simulink model "gm_parallel_lht"  (R2019b)
settings: Solver=FixedStepDiscrete  StartTime=0.0  StopTime=inf  RelTol=1e-3
undefined symbols (not defined in the file or in its folder): bt, height, width
libraries: hdlsllib x190, simulink x13, hdlmdlgenlib x7, dspsrcs4 x1
(part 11 of 18)

== system gm_parallel_lht/Parallel LHT/Parallel LHT Accumulator/Accumulator with Switches/Accumulator_instance41/Block RAM ==
  wr_data : Inport  OutDataTypeStr=fixdt(0, 10, 0)  PortDimensions=1  SampleTime=6.66666666666667e-09
  wr_addr : Inport  Port=2  OutDataTypeStr=fixdt(0, 10, 0)  PortDimensions=1  SampleTime=6.66666666666667e-09
  wr_en : Inport  Port=3  OutDataTypeStr=boolean  PortDimensions=1  SampleTime=6.66666666666667e-09
  rd_addr : Inport  Port=4  OutDataTypeStr=fixdt(0, 10, 0)  PortDimensions=1  SampleTime=6.66666666666667e-09
  Simple Dual Port RAM : Subsystem
  rd_data : Outport
  wires:
  rd_addr/1 -> Simple Dual Port RAM/4(rd_addr)
  wr_en/1 -> Simple Dual Port RAM/3(wr_en)
  wr_addr/1 -> Simple Dual Port RAM/2(wr_addr)
  wr_data/1 -> Simple Dual Port RAM/1(wr_data)
  Simple Dual Port RAM/1(rd_data) -> rd_data/1

== system gm_parallel_lht/Parallel LHT/Parallel LHT Accumulator/Accumulator with Switches/Accumulator_instance42/Block RAM ==
  wr_data : Inport  OutDataTypeStr=fixdt(0, 10, 0)  PortDimensions=1  SampleTime=6.66666666666667e-09
  wr_addr : Inport  Port=2  OutDataTypeStr=fixdt(0, 10, 0)  PortDimensions=1  SampleTime=6.66666666666667e-09
  wr_en : Inport  Port=3  OutDataTypeStr=boolean  PortDimensions=1  SampleTime=6.66666666666667e-09
  rd_addr : Inport  Port=4  OutDataTypeStr=fixdt(0, 10, 0)  PortDimensions=1  SampleTime=6.66666666666667e-09
  Simple Dual Port RAM : Subsystem
  rd_data : Outport
  wires:
  rd_addr/1 -> Simple Dual Port RAM/4(rd_addr)
  wr_en/1 -> Simple Dual Port RAM/3(wr_en)
  wr_addr/1 -> Simple Dual Port RAM/2(wr_addr)
  wr_data/1 -> Simple Dual Port RAM/1(wr_data)
  Simple Dual Port RAM/1(rd_data) -> rd_data/1

== system gm_parallel_lht/Parallel LHT/Parallel LHT Accumulator/Accumulator with Switches/Accumulator_instance43/Block RAM ==
  wr_data : Inport  OutDataTypeStr=fixdt(0, 10, 0)  PortDimensions=1  SampleTime=6.66666666666667e-09
  wr_addr : Inport  Port=2  OutDataTypeStr=fixdt(0, 10, 0)  PortDimensions=1  SampleTime=6.66666666666667e-09
  wr_en : Inport  Port=3  OutDataTypeStr=boolean  PortDimensions=1  SampleTime=6.66666666666667e-09
  rd_addr : Inport  Port=4  OutDataTypeStr=fixdt(0, 10, 0)  PortDimensions=1  SampleTime=6.66666666666667e-09
  Simple Dual Port RAM : Subsystem
  rd_data : Outport
  wires:
  rd_addr/1 -> Simple Dual Port RAM/4(rd_addr)
  wr_en/1 -> Simple Dual Port RAM/3(wr_en)
  wr_addr/1 -> Simple Dual Port RAM/2(wr_addr)
  wr_data/1 -> Simple Dual Port RAM/1(wr_data)
  Simple Dual Port RAM/1(rd_data) -> rd_data/1

== system gm_parallel_lht/Parallel LHT/Parallel LHT Accumulator/Accumulator with Switches/Accumulator_instance44/Block RAM ==
  wr_data : Inport  OutDataTypeStr=fixdt(0, 10, 0)  PortDimensions=1  SampleTime=6.66666666666667e-09
  wr_addr : Inport  Port=2  OutDataTypeStr=fixdt(0, 10, 0)  PortDimensions=1  SampleTime=6.66666666666667e-09
  wr_en : Inport  Port=3  OutDataTypeStr=boolean  PortDimensions=1  SampleTime=6.66666666666667e-09
  rd_addr : Inport  Port=4  OutDataTypeStr=fixdt(0, 10, 0)  PortDimensions=1  SampleTime=6.66666666666667e-09
  Simple Dual Port RAM : Subsystem
  rd_data : Outport
  wires:
  rd_addr/1 -> Simple Dual Port RAM/4(rd_addr)
  wr_en/1 -> Simple Dual Port RAM/3(wr_en)
  wr_addr/1 -> Simple Dual Port RAM/2(wr_addr)
  wr_data/1 -> Simple Dual Port RAM/1(wr_data)
  Simple Dual Port RAM/1(rd_data) -> rd_data/1

== system gm_parallel_lht/Parallel LHT/Parallel LHT Accumulator/Accumulator with Switches/Accumulator_instance45/Block RAM ==
  wr_data : Inport  OutDataTypeStr=fixdt(0, 10, 0)  PortDimensions=1  SampleTime=6.66666666666667e-09
  wr_addr : Inport  Port=2  OutDataTypeStr=fixdt(0, 10, 0)  PortDimensions=1  SampleTime=6.66666666666667e-09
  wr_en : Inport  Port=3  OutDataTypeStr=boolean  PortDimensions=1  SampleTime=6.66666666666667e-09
  rd_addr : Inport  Port=4  OutDataTypeStr=fixdt(0, 10, 0)  PortDimensions=1  SampleTime=6.66666666666667e-09
  Simple Dual Port RAM : Subsystem
  rd_data : Outport
  wires:
  rd_addr/1 -> Simple Dual Port RAM/4(rd_addr)
  wr_en/1 -> Simple Dual Port RAM/3(wr_en)
  wr_addr/1 -> Simple Dual Port RAM/2(wr_addr)
  wr_data/1 -> Simple Dual Port RAM/1(wr_data)
  Simple Dual Port RAM/1(rd_data) -> rd_data/1

== system gm_parallel_lht/Parallel LHT/Parallel LHT Accumulator/Accumulator with Switches/Accumulator_instance46/Block RAM ==
  wr_data : Inport  OutDataTypeStr=fixdt(0, 10, 0)  PortDimensions=1  SampleTime=6.66666666666667e-09
  wr_addr : Inport  Port=2  OutDataTypeStr=fixdt(0, 10, 0)  PortDimensions=1  SampleTime=6.66666666666667e-09
  wr_en : Inport  Port=3  OutDataTypeStr=boolean  PortDimensions=1  SampleTime=6.66666666666667e-09
  rd_addr : Inport  Port=4  OutDataTypeStr=fixdt(0, 10, 0)  PortDimensions=1  SampleTime=6.66666666666667e-09
  Simple Dual Port RAM : Subsystem
  rd_data : Outport
  wires:
  rd_addr/1 -> Simple Dual Port RAM/4(rd_addr)
  wr_en/1 -> Simple Dual Port RAM/3(wr_en)
  wr_addr/1 -> Simple Dual Port RAM/2(wr_addr)
  wr_data/1 -> Simple Dual Port RAM/1(wr_data)
  Simple Dual Port RAM/1(rd_data) -> rd_data/1

== system gm_parallel_lht/Parallel LHT/Parallel LHT Accumulator/Accumulator with Switches/Accumulator_instance47/Block RAM ==
  wr_data : Inport  OutDataTypeStr=fixdt(0, 10, 0)  PortDimensions=1  SampleTime=6.66666666666667e-09
  wr_addr : Inport  Port=2  OutDataTypeStr=fixdt(0, 10, 0)  PortDimensions=1  SampleTime=6.66666666666667e-09
  wr_en : Inport  Port=3  OutDataTypeStr=boolean  PortDimensions=1  SampleTime=6.66666666666667e-09
  rd_addr : Inport  Port=4  OutDataTypeStr=fixdt(0, 10, 0)  PortDimensions=1  SampleTime=6.66666666666667e-09
  Simple Dual Port RAM : Subsystem
  rd_data : Outport
  wires:
  rd_addr/1 -> Simple Dual Port RAM/4(rd_addr)
  wr_en/1 -> Simple Dual Port RAM/3(wr_en)
  wr_addr/1 -> Simple Dual Port RAM/2(wr_addr)
  wr_data/1 -> Simple Dual Port RAM/1(wr_data)
  Simple Dual Port RAM/1(rd_data) -> rd_data/1

== system gm_parallel_lht/Parallel LHT/Parallel LHT Accumulator/Accumulator with Switches/Accumulator_instance48/Block RAM ==
  wr_data : Inport  OutDataTypeStr=fixdt(0, 10, 0)  PortDimensions=1  SampleTime=6.66666666666667e-09
  wr_addr : Inport  Port=2  OutDataTypeStr=fixdt(0, 10, 0)  PortDimensions=1  SampleTime=6.66666666666667e-09
  wr_en : Inport  Port=3  OutDataTypeStr=boolean  PortDimensions=1  SampleTime=6.66666666666667e-09
  rd_addr : Inport  Port=4  OutDataTypeStr=fixdt(0, 10, 0)  PortDimensions=1  SampleTime=6.66666666666667e-09
  Simple Dual Port RAM : Subsystem
  rd_data : Outport
  wires:
  rd_addr/1 -> Simple Dual Port RAM/4(rd_addr)
  wr_en/1 -> Simple Dual Port RAM/3(wr_en)
  wr_addr/1 -> Simple Dual Port RAM/2(wr_addr)
  wr_data/1 -> Simple Dual Port RAM/1(wr_data)
  Simple Dual Port RAM/1(rd_data) -> rd_data/1

== system gm_parallel_lht/Parallel LHT/Parallel LHT Accumulator/Accumulator with Switches/Accumulator_instance49/Block RAM ==
  wr_data : Inport  OutDataTypeStr=fixdt(0, 10, 0)  PortDimensions=1  SampleTime=6.66666666666667e-09
  wr_addr : Inport  Port=2  OutDataTypeStr=fixdt(0, 10, 0)  PortDimensions=1  SampleTime=6.66666666666667e-09
  wr_en : Inport  Port=3  OutDataTypeStr=boolean  PortDimensions=1  SampleTime=6.66666666666667e-09
  rd_addr : Inport  Port=4  OutDataTypeStr=fixdt(0, 10, 0)  PortDimensions=1  SampleTime=6.66666666666667e-09
  Simple Dual Port RAM : Subsystem
  rd_data : Outport
  wires:
  rd_addr/1 -> Simple Dual Port RAM/4(rd_addr)
  wr_en/1 -> Simple Dual Port RAM/3(wr_en)
  wr_addr/1 -> Simple Dual Port RAM/2(wr_addr)
  wr_data/1 -> Simple Dual Port RAM/1(wr_data)
  Simple Dual Port RAM/1(rd_data) -> rd_data/1

== system gm_parallel_lht/Parallel LHT/Parallel LHT Accumulator/Accumulator with Switches/Accumulator_instance5/Block RAM ==
  wr_data : Inport  OutDataTypeStr=fixdt(0, 10, 0)  PortDimensions=1  SampleTime=6.66666666666667e-09
  wr_addr : Inport  Port=2  OutDataTypeStr=fixdt(0, 10, 0)  PortDimensions=1  SampleTime=6.66666666666667e-09
  wr_en : Inport  Port=3  OutDataTypeStr=boolean  PortDimensions=1  SampleTime=6.66666666666667e-09
  rd_addr : Inport  Port=4  OutDataTypeStr=fixdt(0, 10, 0)  PortDimensions=1  SampleTime=6.66666666666667e-09
  Simple Dual Port RAM : Subsystem
  rd_data : Outport
  wires:
  rd_addr/1 -> Simple Dual Port RAM/4(rd_addr)
  wr_en/1 -> Simple Dual Port RAM/3(wr_en)
  wr_addr/1 -> Simple Dual Port RAM/2(wr_addr)
  wr_data/1 -> Simple Dual Port RAM/1(wr_data)
  Simple Dual Port RAM/1(rd_data) -> rd_data/1

== system gm_parallel_lht/Parallel LHT/Parallel LHT Accumulator/Accumulator with Switches/Accumulator_instance50/Block RAM ==
  wr_data : Inport  OutDataTypeStr=fixdt(0, 10, 0)  PortDimensions=1  SampleTime=6.66666666666667e-09
  wr_addr : Inport  Port=2  OutDataTypeStr=fixdt(0, 10, 0)  PortDimensions=1  SampleTime=6.66666666666667e-09
  wr_en : Inport  Port=3  OutDataTypeStr=boolean  PortDimensions=1  SampleTime=6.66666666666667e-09
  rd_addr : Inport  Port=4  OutDataTypeStr=fixdt(0, 10, 0)  PortDimensions=1  SampleTime=6.66666666666667e-09
  Simple Dual Port RAM : Subsystem
  rd_data : Outport
  wires:
  rd_addr/1 -> Simple Dual Port RAM/4(rd_addr)
  wr_en/1 -> Simple Dual Port RAM/3(wr_en)
  wr_addr/1 -> Simple Dual Port RAM/2(wr_addr)
  wr_data/1 -> Simple Dual Port RAM/1(wr_data)
  Simple Dual Port RAM/1(rd_data) -> rd_data/1

== system gm_parallel_lht/Parallel LHT/Parallel LHT Accumulator/Accumulator with Switches/Accumulator_instance51/Block RAM ==
  wr_data : Inport  OutDataTypeStr=fixdt(0, 10, 0)  PortDimensions=1  SampleTime=6.66666666666667e-09
  wr_addr : Inport  Port=2  OutDataTypeStr=fixdt(0, 10, 0)  PortDimensions=1  SampleTime=6.66666666666667e-09
  wr_en : Inport  Port=3  OutDataTypeStr=boolean  PortDimensions=1  SampleTime=6.66666666666667e-09
  rd_addr : Inport  Port=4  OutDataTypeStr=fixdt(0, 10, 0)  PortDimensions=1  SampleTime=6.66666666666667e-09
  Simple Dual Port RAM : Subsystem
  rd_data : Outport
  wires:
  rd_addr/1 -> Simple Dual Port RAM/4(rd_addr)
  wr_en/1 -> Simple Dual Port RAM/3(wr_en)
  wr_addr/1 -> Simple Dual Port RAM/2(wr_addr)
  wr_data/1 -> Simple Dual Port RAM/1(wr_data)
  Simple Dual Port RAM/1(rd_data) -> rd_data/1

== system gm_parallel_lht/Parallel LHT/Parallel LHT Accumulator/Accumulator with Switches/Accumulator_instance52/Block RAM ==
  wr_data : Inport  OutDataTypeStr=fixdt(0, 10, 0)  PortDimensions=1  SampleTime=6.66666666666667e-09
  wr_addr : Inport  Port=2  OutDataTypeStr=fixdt(0, 10, 0)  PortDimensions=1  SampleTime=6.66666666666667e-09
  wr_en : Inport  Port=3  OutDataTypeStr=boolean  PortDimensions=1  SampleTime=6.66666666666667e-09
  rd_addr : Inport  Port=4  OutDataTypeStr=fixdt(0, 10, 0)  PortDimensions=1  SampleTime=6.66666666666667e-09
  Simple Dual Port RAM : Subsystem
  rd_data : Outport
  wires:
  rd_addr/1 -> Simple Dual Port RAM/4(rd_addr)
  wr_en/1 -> Simple Dual Port RAM/3(wr_en)
  wr_addr/1 -> Simple Dual Port RAM/2(wr_addr)
  wr_data/1 -> Simple Dual Port RAM/1(wr_data)
  Simple Dual Port RAM/1(rd_data) -> rd_data/1

== system gm_parallel_lht/Parallel LHT/Parallel LHT Accumulator/Accumulator with Switches/Accumulator_instance53/Block RAM ==
  wr_data : Inport  OutDataTypeStr=fixdt(0, 10, 0)  PortDimensions=1  SampleTime=6.66666666666667e-09
  wr_addr : Inport  Port=2  OutDataTypeStr=fixdt(0, 10, 0)  PortDimensions=1  SampleTime=6.66666666666667e-09
  wr_en : Inport  Port=3  OutDataTypeStr=boolean  PortDimensions=1  SampleTime=6.66666666666667e-09
  rd_addr : Inport  Port=4  OutDataTypeStr=fixdt(0, 10, 0)  PortDimensions=1  SampleTime=6.66666666666667e-09
  Simple Dual Port RAM : Subsystem
  rd_data : Outport
  wires:
  rd_addr/1 -> Simple Dual Port RAM/4(rd_addr)
  wr_en/1 -> Simple Dual Port RAM/3(wr_en)
  wr_addr/1 -> Simple Dual Port RAM/2(wr_addr)
  wr_data/1 -> Simple Dual Port RAM/1(wr_data)
  Simple Dual Port RAM/1(rd_data) -> rd_data/1

== system gm_parallel_lht/Parallel LHT/Parallel LHT Accumulator/Accumulator with Switches/Accumulator_instance54/Block RAM ==
  wr_data : Inport  OutDataTypeStr=fixdt(0, 10, 0)  PortDimensions=1  SampleTime=6.66666666666667e-09
  wr_addr : Inport  Port=2  OutDataTypeStr=fixdt(0, 10, 0)  PortDimensions=1  SampleTime=6.66666666666667e-09
  wr_en : Inport  Port=3  OutDataTypeStr=boolean  PortDimensions=1  SampleTime=6.66666666666667e-09
  rd_addr : Inport  Port=4  OutDataTypeStr=fixdt(0, 10, 0)  PortDimensions=1  SampleTime=6.66666666666667e-09
  Simple Dual Port RAM : Subsystem
  rd_data : Outport
  wires:
  rd_addr/1 -> Simple Dual Port RAM/4(rd_addr)
  wr_en/1 -> Simple Dual Port RAM/3(wr_en)
  wr_addr/1 -> Simple Dual Port RAM/2(wr_addr)
  wr_data/1 -> Simple Dual Port RAM/1(wr_data)
  Simple Dual Port RAM/1(rd_data) -> rd_data/1

== system gm_parallel_lht/Parallel LHT/Parallel LHT Accumulator/Accumulator with Switches/Accumulator_instance55/Block RAM ==
  wr_data : Inport  OutDataTypeStr=fixdt(0, 10, 0)  PortDimensions=1  SampleTime=6.66666666666667e-09
  wr_addr : Inport  Port=2  OutDataTypeStr=fixdt(0, 10, 0)  PortDimensions=1  SampleTime=6.66666666666667e-09
  wr_en : Inport  Port=3  OutDataTypeStr=boolean  PortDimensions=1  SampleTime=6.66666666666667e-09
  rd_addr : Inport  Port=4  OutDataTypeStr=fixdt(0, 10, 0)  PortDimensions=1  SampleTime=6.66666666666667e-09
  Simple Dual Port RAM : Subsystem
  rd_data : Outport
  wires:
  rd_addr/1 -> Simple Dual Port RAM/4(rd_addr)
  wr_en/1 -> Simple Dual Port RAM/3(wr_en)
  wr_addr/1 -> Simple Dual Port RAM/2(wr_addr)
  wr_data/1 -> Simple Dual Port RAM/1(wr_data)
  Simple Dual Port RAM/1(rd_data) -> rd_data/1

== system gm_parallel_lht/Parallel LHT/Parallel LHT Accumulator/Accumulator with Switches/Accumulator_instance56/Block RAM ==
  wr_data : Inport  OutDataTypeStr=fixdt(0, 10, 0)  PortDimensions=1  SampleTime=6.66666666666667e-09
  wr_addr : Inport  Port=2  OutDataTypeStr=fixdt(0, 10, 0)  PortDimensions=1  SampleTime=6.66666666666667e-09
  wr_en : Inport  Port=3  OutDataTypeStr=boolean  PortDimensions=1  SampleTime=6.66666666666667e-09
  rd_addr : Inport  Port=4  OutDataTypeStr=fixdt(0, 10, 0)  PortDimensions=1  SampleTime=6.66666666666667e-09
  Simple Dual Port RAM : Subsystem
  rd_data : Outport
  wires:
  rd_addr/1 -> Simple Dual Port RAM/4(rd_addr)
  wr_en/1 -> Simple Dual Port RAM/3(wr_en)
  wr_addr/1 -> Simple Dual Port RAM/2(wr_addr)
  wr_data/1 -> Simple Dual Port RAM/1(wr_data)
  Simple Dual Port RAM/1(rd_data) -> rd_data/1

== system gm_parallel_lht/Parallel LHT/Parallel LHT Accumulator/Accumulator with Switches/Accumulator_instance57/Block RAM ==
  wr_data : Inport  OutDataTypeStr=fixdt(0, 10, 0)  PortDimensions=1  SampleTime=6.66666666666667e-09
  wr_addr : Inport  Port=2  OutDataTypeStr=fixdt(0, 10, 0)  PortDimensions=1  SampleTime=6.66666666666667e-09
  wr_en : Inport  Port=3  OutDataTypeStr=boolean  PortDimensions=1  SampleTime=6.66666666666667e-09
  rd_addr : Inport  Port=4  OutDataTypeStr=fixdt(0, 10, 0)  PortDimensions=1  SampleTime=6.66666666666667e-09
  Simple Dual Port RAM : Subsystem
  rd_data : Outport
  wires:
  rd_addr/1 -> Simple Dual Port RAM/4(rd_addr)
  wr_en/1 -> Simple Dual Port RAM/3(wr_en)
  wr_addr/1 -> Simple Dual Port RAM/2(wr_addr)
  wr_data/1 -> Simple Dual Port RAM/1(wr_data)
  Simple Dual Port RAM/1(rd_data) -> rd_data/1

== system gm_parallel_lht/Parallel LHT/Parallel LHT Accumulator/Accumulator with Switches/Accumulator_instance58/Block RAM ==
  wr_data : Inport  OutDataTypeStr=fixdt(0, 10, 0)  PortDimensions=1  SampleTime=6.66666666666667e-09
  wr_addr : Inport  Port=2  OutDataTypeStr=fixdt(0, 10, 0)  PortDimensions=1  SampleTime=6.66666666666667e-09
  wr_en : Inport  Port=3  OutDataTypeStr=boolean  PortDimensions=1  SampleTime=6.66666666666667e-09
  rd_addr : Inport  Port=4  OutDataTypeStr=fixdt(0, 10, 0)  PortDimensions=1  SampleTime=6.66666666666667e-09
  Simple Dual Port RAM : Subsystem
  rd_data : Outport
  wires:
  rd_addr/1 -> Simple Dual Port RAM/4(rd_addr)
  wr_en/1 -> Simple Dual Port RAM/3(wr_en)
  wr_addr/1 -> Simple Dual Port RAM/2(wr_addr)
  wr_data/1 -> Simple Dual Port RAM/1(wr_data)
  Simple Dual Port RAM/1(rd_data) -> rd_data/1

== system gm_parallel_lht/Parallel LHT/Parallel LHT Accumulator/Accumulator with Switches/Accumulator_instance59/Block RAM ==
  wr_data : Inport  OutDataTypeStr=fixdt(0, 10, 0)  PortDimensions=1  SampleTime=6.66666666666667e-09
  wr_addr : Inport  Port=2  OutDataTypeStr=fixdt(0, 10, 0)  PortDimensions=1  SampleTime=6.66666666666667e-09
  wr_en : Inport  Port=3  OutDataTypeStr=boolean  PortDimensions=1  SampleTime=6.66666666666667e-09
  rd_addr : Inport  Port=4  OutDataTypeStr=fixdt(0, 10, 0)  PortDimensions=1  SampleTime=6.66666666666667e-09
  Simple Dual Port RAM : Subsystem
  rd_data : Outport
  wires:
  rd_addr/1 -> Simple Dual Port RAM/4(rd_addr)
  wr_en/1 -> Simple Dual Port RAM/3(wr_en)
  wr_addr/1 -> Simple Dual Port RAM/2(wr_addr)
  wr_data/1 -> Simple Dual Port RAM/1(wr_data)
  Simple Dual Port RAM/1(rd_data) -> rd_data/1

== system gm_parallel_lht/Parallel LHT/Parallel LHT Accumulator/Accumulator with Switches/Accumulator_instance6/Block RAM ==
  wr_data : Inport  OutDataTypeStr=fixdt(0, 10, 0)  PortDimensions=1  SampleTime=6.66666666666667e-09
  wr_addr : Inport  Port=2  OutDataTypeStr=fixdt(0, 10, 0)  PortDimensions=1  SampleTime=6.66666666666667e-09
  wr_en : Inport  Port=3  OutDataTypeStr=boolean  PortDimensions=1  SampleTime=6.66666666666667e-09
  rd_addr : Inport  Port=4  OutDataTypeStr=fixdt(0, 10, 0)  PortDimensions=1  SampleTime=6.66666666666667e-09
  Simple Dual Port RAM : Subsystem
  rd_data : Outport
  wires:
  rd_addr/1 -> Simple Dual Port RAM/4(rd_addr)
  wr_en/1 -> Simple Dual Port RAM/3(wr_en)
  wr_addr/1 -> Simple Dual Port RAM/2(wr_addr)
  wr_data/1 -> Simple Dual Port RAM/1(wr_data)
  Simple Dual Port RAM/1(rd_data) -> rd_data/1

== system gm_parallel_lht/Parallel LHT/Parallel LHT Accumulator/Accumulator with Switches/Accumulator_instance60/Block RAM ==
  wr_data : Inport  OutDataTypeStr=fixdt(0, 10, 0)  PortDimensions=1  SampleTime=6.66666666666667e-09
  wr_addr : Inport  Port=2  OutDataTypeStr=fixdt(0, 10, 0)  PortDimensions=1  SampleTime=6.66666666666667e-09
  wr_en : Inport  Port=3  OutDataTypeStr=boolean  PortDimensions=1  SampleTime=6.66666666666667e-09
  rd_addr : Inport  Port=4  OutDataTypeStr=fixdt(0, 10, 0)  PortDimensions=1  SampleTime=6.66666666666667e-09
  Simple Dual Port RAM : Subsystem
  rd_data : Outport
  wires:
  rd_addr/1 -> Simple Dual Port RAM/4(rd_addr)
  wr_en/1 -> Simple Dual Port RAM/3(wr_en)
  wr_addr/1 -> Simple Dual Port RAM/2(wr_addr)
  wr_data/1 -> Simple Dual Port RAM/1(wr_data)
  Simple Dual Port RAM/1(rd_data) -> rd_data/1

== system gm_parallel_lht/Parallel LHT/Parallel LHT Accumulator/Accumulator with Switches/Accumulator_instance61/Block RAM ==
  wr_data : Inport  OutDataTypeStr=fixdt(0, 10, 0)  PortDimensions=1  SampleTime=6.66666666666667e-09
  wr_addr : Inport  Port=2  OutDataTypeStr=fixdt(0, 10, 0)  PortDimensions=1  SampleTime=6.66666666666667e-09
  wr_en : Inport  Port=3  OutDataTypeStr=boolean  PortDimensions=1  SampleTime=6.66666666666667e-09
  rd_addr : Inport  Port=4  OutDataTypeStr=fixdt(0, 10, 0)  PortDimensions=1  SampleTime=6.66666666666667e-09
  Simple Dual Port RAM : Subsystem
  rd_data : Outport
  wires:
  rd_addr/1 -> Simple Dual Port RAM/4(rd_addr)
  wr_en/1 -> Simple Dual Port RAM/3(wr_en)
  wr_addr/1 -> Simple Dual Port RAM/2(wr_addr)
  wr_data/1 -> Simple Dual Port RAM/1(wr_data)
  Simple Dual Port RAM/1(rd_data) -> rd_data/1

== system gm_parallel_lht/Parallel LHT/Parallel LHT Accumulator/Accumulator with Switches/Accumulator_instance62/Block RAM ==
  wr_data : Inport  OutDataTypeStr=fixdt(0, 10, 0)  PortDimensions=1  SampleTime=6.66666666666667e-09
  wr_addr : Inport  Port=2  OutDataTypeStr=fixdt(0, 10, 0)  PortDimensions=1  SampleTime=6.66666666666667e-09
  wr_en : Inport  Port=3  OutDataTypeStr=boolean  PortDimensions=1  SampleTime=6.66666666666667e-09
  rd_addr : Inport  Port=4  OutDataTypeStr=fixdt(0, 10, 0)  PortDimensions=1  SampleTime=6.66666666666667e-09
  Simple Dual Port RAM : Subsystem
  rd_data : Outport
  wires:
  rd_addr/1 -> Simple Dual Port RAM/4(rd_addr)
  wr_en/1 -> Simple Dual Port RAM/3(wr_en)
  wr_addr/1 -> Simple Dual Port RAM/2(wr_addr)
  wr_data/1 -> Simple Dual Port RAM/1(wr_data)
  Simple Dual Port RAM/1(rd_data) -> rd_data/1

== system gm_parallel_lht/Parallel LHT/Parallel LHT Accumulator/Accumulator with Switches/Accumulator_instance63/Block RAM ==
  wr_data : Inport  OutDataTypeStr=fixdt(0, 10, 0)  PortDimensions=1  SampleTime=6.66666666666667e-09
  wr_addr : Inport  Port=2  OutDataTypeStr=fixdt(0, 10, 0)  PortDimensions=1  SampleTime=6.66666666666667e-09
  wr_en : Inport  Port=3  OutDataTypeStr=boolean  PortDimensions=1  SampleTime=6.66666666666667e-09
  rd_addr : Inport  Port=4  OutDataTypeStr=fixdt(0, 10, 0)  PortDimensions=1  SampleTime=6.66666666666667e-09
  Simple Dual Port RAM : Subsystem
  rd_data : Outport
  wires:
  rd_addr/1 -> Simple Dual Port RAM/4(rd_addr)
  wr_en/1 -> Simple Dual Port RAM/3(wr_en)
  wr_addr/1 -> Simple Dual Port RAM/2(wr_addr)
  wr_data/1 -> Simple Dual Port RAM/1(wr_data)
  Simple Dual Port RAM/1(rd_data) -> rd_data/1

== system gm_parallel_lht/Parallel LHT/Parallel LHT Accumulator/Accumulator with Switches/Accumulator_instance64/Block RAM ==
  wr_data : Inport  OutDataTypeStr=fixdt(0, 10, 0)  PortDimensions=1  SampleTime=6.66666666666667e-09
  wr_addr : Inport  Port=2  OutDataTypeStr=fixdt(0, 10, 0)  PortDimensions=1  SampleTime=6.66666666666667e-09
  wr_en : Inport  Port=3  OutDataTypeStr=boolean  PortDimensions=1  SampleTime=6.66666666666667e-09
  rd_addr : Inport  Port=4  OutDataTypeStr=fixdt(0, 10, 0)  PortDimensions=1  SampleTime=6.66666666666667e-09
  Simple Dual Port RAM : Subsystem
  rd_data : Outport
  wires:
  rd_addr/1 -> Simple Dual Port RAM/4(rd_addr)
  wr_en/1 -> Simple Dual Port RAM/3(wr_en)
  wr_addr/1 -> Simple Dual Port RAM/2(wr_addr)
  wr_data/1 -> Simple Dual Port RAM/1(wr_data)
  Simple Dual Port RAM/1(rd_data) -> rd_data/1

== system gm_parallel_lht/Parallel LHT/Parallel LHT Accumulator/Accumulator with Switches/Accumulator_instance65/Block RAM ==
  wr_data : Inport  OutDataTypeStr=fixdt(0, 10, 0)  PortDimensions=1  SampleTime=6.66666666666667e-09
  wr_addr : Inport  Port=2  OutDataTypeStr=fixdt(0, 10, 0)  PortDimensions=1  SampleTime=6.66666666666667e-09
  wr_en : Inport  Port=3  OutDataTypeStr=boolean  PortDimensions=1  SampleTime=6.66666666666667e-09
  rd_addr : Inport  Port=4  OutDataTypeStr=fixdt(0, 10, 0)  PortDimensions=1  SampleTime=6.66666666666667e-09
  Simple Dual Port RAM : Subsystem
  rd_data : Outport
  wires:
  rd_addr/1 -> Simple Dual Port RAM/4(rd_addr)
  wr_en/1 -> Simple Dual Port RAM/3(wr_en)
  wr_addr/1 -> Simple Dual Port RAM/2(wr_addr)
  wr_data/1 -> Simple Dual Port RAM/1(wr_data)
  Simple Dual Port RAM/1(rd_data) -> rd_data/1

== system gm_parallel_lht/Parallel LHT/Parallel LHT Accumulator/Accumulator with Switches/Accumulator_instance66/Block RAM ==
  wr_data : Inport  OutDataTypeStr=fixdt(0, 10, 0)  PortDimensions=1  SampleTime=6.66666666666667e-09
  wr_addr : Inport  Port=2  OutDataTypeStr=fixdt(0, 10, 0)  PortDimensions=1  SampleTime=6.66666666666667e-09
  wr_en : Inport  Port=3  OutDataTypeStr=boolean  PortDimensions=1  SampleTime=6.66666666666667e-09
  rd_addr : Inport  Port=4  OutDataTypeStr=fixdt(0, 10, 0)  PortDimensions=1  SampleTime=6.66666666666667e-09
  Simple Dual Port RAM : Subsystem
  rd_data : Outport
  wires:
  rd_addr/1 -> Simple Dual Port RAM/4(rd_addr)
  wr_en/1 -> Simple Dual Port RAM/3(wr_en)
  wr_addr/1 -> Simple Dual Port RAM/2(wr_addr)
  wr_data/1 -> Simple Dual Port RAM/1(wr_data)
  Simple Dual Port RAM/1(rd_data) -> rd_data/1

== system gm_parallel_lht/Parallel LHT/Parallel LHT Accumulator/Accumulator with Switches/Accumulator_instance67/Block RAM ==
  wr_data : Inport  OutDataTypeStr=fixdt(0, 10, 0)  PortDimensions=1  SampleTime=6.66666666666667e-09
  wr_addr : Inport  Port=2  OutDataTypeStr=fixdt(0, 10, 0)  PortDimensions=1  SampleTime=6.66666666666667e-09
  wr_en : Inport  Port=3  OutDataTypeStr=boolean  PortDimensions=1  SampleTime=6.66666666666667e-09
  rd_addr : Inport  Port=4  OutDataTypeStr=fixdt(0, 10, 0)  PortDimensions=1  SampleTime=6.66666666666667e-09
  Simple Dual Port RAM : Subsystem
  rd_data : Outport
  wires:
  rd_addr/1 -> Simple Dual Port RAM/4(rd_addr)
  wr_en/1 -> Simple Dual Port RAM/3(wr_en)
  wr_addr/1 -> Simple Dual Port RAM/2(wr_addr)
  wr_data/1 -> Simple Dual Port RAM/1(wr_data)
  Simple Dual Port RAM/1(rd_data) -> rd_data/1

== system gm_parallel_lht/Parallel LHT/Parallel LHT Accumulator/Accumulator with Switches/Accumulator_instance68/Block RAM ==
  wr_data : Inport  OutDataTypeStr=fixdt(0, 10, 0)  PortDimensions=1  SampleTime=6.66666666666667e-09
  wr_addr : Inport  Port=2  OutDataTypeStr=fixdt(0, 10, 0)  PortDimensions=1  SampleTime=6.66666666666667e-09
  wr_en : Inport  Port=3  OutDataTypeStr=boolean  PortDimensions=1  SampleTime=6.66666666666667e-09
  rd_addr : Inport  Port=4  OutDataTypeStr=fixdt(0, 10, 0)  PortDimensions=1  SampleTime=6.66666666666667e-09
  Simple Dual Port RAM : Subsystem
  rd_data : Outport
  wires:
  rd_addr/1 -> Simple Dual Port RAM/4(rd_addr)
  wr_en/1 -> Simple Dual Port RAM/3(wr_en)
  wr_addr/1 -> Simple Dual Port RAM/2(wr_addr)
  wr_data/1 -> Simple Dual Port RAM/1(wr_data)
  Simple Dual Port RAM/1(rd_data) -> rd_data/1

== system gm_parallel_lht/Parallel LHT/Parallel LHT Accumulator/Accumulator with Switches/Accumulator_instance69/Block RAM ==
  wr_data : Inport  OutDataTypeStr=fixdt(0, 10, 0)  PortDimensions=1  SampleTime=6.66666666666667e-09
  wr_addr : Inport  Port=2  OutDataTypeStr=fixdt(0, 10, 0)  PortDimensions=1  SampleTime=6.66666666666667e-09
  wr_en : Inport  Port=3  OutDataTypeStr=boolean  PortDimensions=1  SampleTime=6.66666666666667e-09
  rd_addr : Inport  Port=4  OutDataTypeStr=fixdt(0, 10, 0)  PortDimensions=1  SampleTime=6.66666666666667e-09
  Simple Dual Port RAM : Subsystem
  rd_data : Outport
  wires:
  rd_addr/1 -> Simple Dual Port RAM/4(rd_addr)
  wr_en/1 -> Simple Dual Port RAM/3(wr_en)
  wr_addr/1 -> Simple Dual Port RAM/2(wr_addr)
  wr_data/1 -> Simple Dual Port RAM/1(wr_data)
  Simple Dual Port RAM/1(rd_data) -> rd_data/1

== system gm_parallel_lht/Parallel LHT/Parallel LHT Accumulator/Accumulator with Switches/Accumulator_instance7/Block RAM ==
  wr_data : Inport  OutDataTypeStr=fixdt(0, 10, 0)  PortDimensions=1  SampleTime=6.66666666666667e-09
  wr_addr : Inport  Port=2  OutDataTypeStr=fixdt(0, 10, 0)  PortDimensions=1  SampleTime=6.66666666666667e-09
  wr_en : Inport  Port=3  OutDataTypeStr=boolean  PortDimensions=1  SampleTime=6.66666666666667e-09
  rd_addr : Inport  Port=4  OutDataTypeStr=fixdt(0, 10, 0)  PortDimensions=1  SampleTime=6.66666666666667e-09
  Simple Dual Port RAM : Subsystem
  rd_data : Outport
  wires:
  rd_addr/1 -> Simple Dual Port RAM/4(rd_addr)
  wr_en/1 -> Simple Dual Port RAM/3(wr_en)
  wr_addr/1 -> Simple Dual Port RAM/2(wr_addr)
  wr_data/1 -> Simple Dual Port RAM/1(wr_data)
  Simple Dual Port RAM/1(rd_data) -> rd_data/1

== system gm_parallel_lht/Parallel LHT/Parallel LHT Accumulator/Accumulator with Switches/Accumulator_instance70/Block RAM ==
  wr_data : Inport  OutDataTypeStr=fixdt(0, 10, 0)  PortDimensions=1  SampleTime=6.66666666666667e-09
  wr_addr : Inport  Port=2  OutDataTypeStr=fixdt(0, 10, 0)  PortDimensions=1  SampleTime=6.66666666666667e-09
  wr_en : Inport  Port=3  OutDataTypeStr=boolean  PortDimensions=1  SampleTime=6.66666666666667e-09
  rd_addr : Inport  Port=4  OutDataTypeStr=fixdt(0, 10, 0)  PortDimensions=1  SampleTime=6.66666666666667e-09
  Simple Dual Port RAM : Subsystem
  rd_data : Outport
  wires:
  rd_addr/1 -> Simple Dual Port RAM/4(rd_addr)
  wr_en/1 -> Simple Dual Port RAM/3(wr_en)
  wr_addr/1 -> Simple Dual Port RAM/2(wr_addr)
  wr_data/1 -> Simple Dual Port RAM/1(wr_data)
  Simple Dual Port RAM/1(rd_data) -> rd_data/1

== system gm_parallel_lht/Parallel LHT/Parallel LHT Accumulator/Accumulator with Switches/Accumulator_instance71/Block RAM ==
  wr_data : Inport  OutDataTypeStr=fixdt(0, 10, 0)  PortDimensions=1  SampleTime=6.66666666666667e-09
  wr_addr : Inport  Port=2  OutDataTypeStr=fixdt(0, 10, 0)  PortDimensions=1  SampleTime=6.66666666666667e-09
  wr_en : Inport  Port=3  OutDataTypeStr=boolean  PortDimensions=1  SampleTime=6.66666666666667e-09
  rd_addr : Inport  Port=4  OutDataTypeStr=fixdt(0, 10, 0)  PortDimensions=1  SampleTime=6.66666666666667e-09
  Simple Dual Port RAM : Subsystem
  rd_data : Outport
  wires:
  rd_addr/1 -> Simple Dual Port RAM/4(rd_addr)
  wr_en/1 -> Simple Dual Port RAM/3(wr_en)
  wr_addr/1 -> Simple Dual Port RAM/2(wr_addr)
  wr_data/1 -> Simple Dual Port RAM/1(wr_data)
  Simple Dual Port RAM/1(rd_data) -> rd_data/1

== system gm_parallel_lht/Parallel LHT/Parallel LHT Accumulator/Accumulator with Switches/Accumulator_instance72/Block RAM ==
  wr_data : Inport  OutDataTypeStr=fixdt(0, 10, 0)  PortDimensions=1  SampleTime=6.66666666666667e-09
  wr_addr : Inport  Port=2  OutDataTypeStr=fixdt(0, 10, 0)  PortDimensions=1  SampleTime=6.66666666666667e-09
  wr_en : Inport  Port=3  OutDataTypeStr=boolean  PortDimensions=1  SampleTime=6.66666666666667e-09
  rd_addr : Inport  Port=4  OutDataTypeStr=fixdt(0, 10, 0)  PortDimensions=1  SampleTime=6.66666666666667e-09
  Simple Dual Port RAM : Subsystem
  rd_data : Outport
  wires:
  rd_addr/1 -> Simple Dual Port RAM/4(rd_addr)
  wr_en/1 -> Simple Dual Port RAM/3(wr_en)
  wr_addr/1 -> Simple Dual Port RAM/2(wr_addr)
  wr_data/1 -> Simple Dual Port RAM/1(wr_data)
  Simple Dual Port RAM/1(rd_data) -> rd_data/1

== system gm_parallel_lht/Parallel LHT/Parallel LHT Accumulator/Accumulator with Switches/Accumulator_instance73/Block RAM ==
  wr_data : Inport  OutDataTypeStr=fixdt(0, 10, 0)  PortDimensions=1  SampleTime=6.66666666666667e-09
  wr_addr : Inport  Port=2  OutDataTypeStr=fixdt(0, 10, 0)  PortDimensions=1  SampleTime=6.66666666666667e-09
  wr_en : Inport  Port=3  OutDataTypeStr=boolean  PortDimensions=1  SampleTime=6.66666666666667e-09
  rd_addr : Inport  Port=4  OutDataTypeStr=fixdt(0, 10, 0)  PortDimensions=1  SampleTime=6.66666666666667e-09
  Simple Dual Port RAM : Subsystem
  rd_data : Outport
  wires:
  rd_addr/1 -> Simple Dual Port RAM/4(rd_addr)
  wr_en/1 -> Simple Dual Port RAM/3(wr_en)
  wr_addr/1 -> Simple Dual Port RAM/2(wr_addr)
  wr_data/1 -> Simple Dual Port RAM/1(wr_data)
  Simple Dual Port RAM/1(rd_data) -> rd_data/1

== system gm_parallel_lht/Parallel LHT/Parallel LHT Accumulator/Accumulator with Switches/Accumulator_instance74/Block RAM ==
  wr_data : Inport  OutDataTypeStr=fixdt(0, 10, 0)  PortDimensions=1  SampleTime=6.66666666666667e-09
  wr_addr : Inport  Port=2  OutDataTypeStr=fixdt(0, 10, 0)  PortDimensions=1  SampleTime=6.66666666666667e-09
  wr_en : Inport  Port=3  OutDataTypeStr=boolean  PortDimensions=1  SampleTime=6.66666666666667e-09
  rd_addr : Inport  Port=4  OutDataTypeStr=fixdt(0, 10, 0)  PortDimensions=1  SampleTime=6.66666666666667e-09
  Simple Dual Port RAM : Subsystem
  rd_data : Outport
  wires:
  rd_addr/1 -> Simple Dual Port RAM/4(rd_addr)
  wr_en/1 -> Simple Dual Port RAM/3(wr_en)
  wr_addr/1 -> Simple Dual Port RAM/2(wr_addr)
  wr_data/1 -> Simple Dual Port RAM/1(wr_data)
  Simple Dual Port RAM/1(rd_data) -> rd_data/1

== system gm_parallel_lht/Parallel LHT/Parallel LHT Accumulator/Accumulator with Switches/Accumulator_instance75/Block RAM ==
  wr_data : Inport  OutDataTypeStr=fixdt(0, 10, 0)  PortDimensions=1  SampleTime=6.66666666666667e-09
  wr_addr : Inport  Port=2  OutDataTypeStr=fixdt(0, 10, 0)  PortDimensions=1  SampleTime=6.66666666666667e-09
  wr_en : Inport  Port=3  OutDataTypeStr=boolean  PortDimensions=1  SampleTime=6.66666666666667e-09
  rd_addr : Inport  Port=4  OutDataTypeStr=fixdt(0, 10, 0)  PortDimensions=1  SampleTime=6.66666666666667e-09
  Simple Dual Port RAM : Subsystem
  rd_data : Outport
  wires:
  rd_addr/1 -> Simple Dual Port RAM/4(rd_addr)
  wr_en/1 -> Simple Dual Port RAM/3(wr_en)
  wr_addr/1 -> Simple Dual Port RAM/2(wr_addr)
  wr_data/1 -> Simple Dual Port RAM/1(wr_data)
  Simple Dual Port RAM/1(rd_data) -> rd_data/1

== system gm_parallel_lht/Parallel LHT/Parallel LHT Accumulator/Accumulator with Switches/Accumulator_instance76/Block RAM ==
  wr_data : Inport  OutDataTypeStr=fixdt(0, 10, 0)  PortDimensions=1  SampleTime=6.66666666666667e-09
  wr_addr : Inport  Port=2  OutDataTypeStr=fixdt(0, 10, 0)  PortDimensions=1  SampleTime=6.66666666666667e-09
  wr_en : Inport  Port=3  OutDataTypeStr=boolean  PortDimensions=1  SampleTime=6.66666666666667e-09
  rd_addr : Inport  Port=4  OutDataTypeStr=fixdt(0, 10, 0)  PortDimensions=1  SampleTime=6.66666666666667e-09
  Simple Dual Port RAM : Subsystem
  rd_data : Outport
  wires:
  rd_addr/1 -> Simple Dual Port RAM/4(rd_addr)
  wr_en/1 -> Simple Dual Port RAM/3(wr_en)
  wr_addr/1 -> Simple Dual Port RAM/2(wr_addr)
  wr_data/1 -> Simple Dual Port RAM/1(wr_data)
  Simple Dual Port RAM/1(rd_data) -> rd_data/1

== system gm_parallel_lht/Parallel LHT/Parallel LHT Accumulator/Accumulator with Switches/Accumulator_instance77/Block RAM ==
  wr_data : Inport  OutDataTypeStr=fixdt(0, 10, 0)  PortDimensions=1  SampleTime=6.66666666666667e-09
  wr_addr : Inport  Port=2  OutDataTypeStr=fixdt(0, 10, 0)  PortDimensions=1  SampleTime=6.66666666666667e-09
  wr_en : Inport  Port=3  OutDataTypeStr=boolean  PortDimensions=1  SampleTime=6.66666666666667e-09
  rd_addr : Inport  Port=4  OutDataTypeStr=fixdt(0, 10, 0)  PortDimensions=1  SampleTime=6.66666666666667e-09
  Simple Dual Port RAM : Subsystem
  rd_data : Outport
  wires:
  rd_addr/1 -> Simple Dual Port RAM/4(rd_addr)
  wr_en/1 -> Simple Dual Port RAM/3(wr_en)
  wr_addr/1 -> Simple Dual Port RAM/2(wr_addr)
  wr_data/1 -> Simple Dual Port RAM/1(wr_data)
  Simple Dual Port RAM/1(rd_data) -> rd_data/1

== system gm_parallel_lht/Parallel LHT/Parallel LHT Accumulator/Accumulator with Switches/Accumulator_instance78/Block RAM ==
  wr_data : Inport  OutDataTypeStr=fixdt(0, 10, 0)  PortDimensions=1  SampleTime=6.66666666666667e-09
  wr_addr : Inport  Port=2  OutDataTypeStr=fixdt(0, 10, 0)  PortDimensions=1  SampleTime=6.66666666666667e-09
  wr_en : Inport  Port=3  OutDataTypeStr=boolean  PortDimensions=1  SampleTime=6.66666666666667e-09
  rd_addr : Inport  Port=4  OutDataTypeStr=fixdt(0, 10, 0)  PortDimensions=1  SampleTime=6.66666666666667e-09
  Simple Dual Port RAM : Subsystem
  rd_data : Outport
  wires:
  rd_addr/1 -> Simple Dual Port RAM/4(rd_addr)
  wr_en/1 -> Simple Dual Port RAM/3(wr_en)
  wr_addr/1 -> Simple Dual Port RAM/2(wr_addr)
  wr_data/1 -> Simple Dual Port RAM/1(wr_data)
  Simple Dual Port RAM/1(rd_data) -> rd_data/1

== system gm_parallel_lht/Parallel LHT/Parallel LHT Accumulator/Accumulator with Switches/Accumulator_instance79/Block RAM ==
  wr_data : Inport  OutDataTypeStr=fixdt(0, 10, 0)  PortDimensions=1  SampleTime=6.66666666666667e-09
  wr_addr : Inport  Port=2  OutDataTypeStr=fixdt(0, 10, 0)  PortDimensions=1  SampleTime=6.66666666666667e-09
  wr_en : Inport  Port=3  OutDataTypeStr=boolean  PortDimensions=1  SampleTime=6.66666666666667e-09
  rd_addr : Inport  Port=4  OutDataTypeStr=fixdt(0, 10, 0)  PortDimensions=1  SampleTime=6.66666666666667e-09
  Simple Dual Port RAM : Subsystem
  rd_data : Outport
  wires:
  rd_addr/1 -> Simple Dual Port RAM/4(rd_addr)
  wr_en/1 -> Simple Dual Port RAM/3(wr_en)
  wr_addr/1 -> Simple Dual Port RAM/2(wr_addr)
  wr_data/1 -> Simple Dual Port RAM/1(wr_data)
  Simple Dual Port RAM/1(rd_data) -> rd_data/1

== system gm_parallel_lht/Parallel LHT/Parallel LHT Accumulator/Accumulator with Switches/Accumulator_instance8/Block RAM ==
  wr_data : Inport  OutDataTypeStr=fixdt(0, 10, 0)  PortDimensions=1  SampleTime=6.66666666666667e-09
  wr_addr : Inport  Port=2  OutDataTypeStr=fixdt(0, 10, 0)  PortDimensions=1  SampleTime=6.66666666666667e-09
  wr_en : Inport  Port=3  OutDataTypeStr=boolean  PortDimensions=1  SampleTime=6.66666666666667e-09
  rd_addr : Inport  Port=4  OutDataTypeStr=fixdt(0, 10, 0)  PortDimensions=1  SampleTime=6.66666666666667e-09
  Simple Dual Port RAM : Subsystem
  rd_data : Outport
  wires:
  rd_addr/1 -> Simple Dual Port RAM/4(rd_addr)
  wr_en/1 -> Simple Dual Port RAM/3(wr_en)
  wr_addr/1 -> Simple Dual Port RAM/2(wr_addr)
  wr_data/1 -> Simple Dual Port RAM/1(wr_data)
  Simple Dual Port RAM/1(rd_data) -> rd_data/1

== system gm_parallel_lht/Parallel LHT/Parallel LHT Accumulator/Accumulator with Switches/Accumulator_instance80/Block RAM ==
  wr_data : Inport  OutDataTypeStr=fixdt(0, 10, 0)  PortDimensions=1  SampleTime=6.66666666666667e-09
  wr_addr : Inport  Port=2  OutDataTypeStr=fixdt(0, 10, 0)  PortDimensions=1  SampleTime=6.66666666666667e-09
  wr_en : Inport  Port=3  OutDataTypeStr=boolean  PortDimensions=1  SampleTime=6.66666666666667e-09
  rd_addr : Inport  Port=4  OutDataTypeStr=fixdt(0, 10, 0)  PortDimensions=1  SampleTime=6.66666666666667e-09
  Simple Dual Port RAM : Subsystem
  rd_data : Outport
  wires:
  rd_addr/1 -> Simple Dual Port RAM/4(rd_addr)
  wr_en/1 -> Simple Dual Port RAM/3(wr_en)
  wr_addr/1 -> Simple Dual Port RAM/2(wr_addr)
  wr_data/1 -> Simple Dual Port RAM/1(wr_data)
  Simple Dual Port RAM/1(rd_data) -> rd_data/1

== system gm_parallel_lht/Parallel LHT/Parallel LHT Accumulator/Accumulator with Switches/Accumulator_instance81/Block RAM ==
  wr_data : Inport  OutDataTypeStr=fixdt(0, 10, 0)  PortDimensions=1  SampleTime=6.66666666666667e-09
  wr_addr : Inport  Port=2  OutDataTypeStr=fixdt(0, 10, 0)  PortDimensions=1  SampleTime=6.66666666666667e-09
  wr_en : Inport  Port=3  OutDataTypeStr=boolean  PortDimensions=1  SampleTime=6.66666666666667e-09
  rd_addr : Inport  Port=4  OutDataTypeStr=fixdt(0, 10, 0)  PortDimensions=1  SampleTime=6.66666666666667e-09
  Simple Dual Port RAM : Subsystem
  rd_data : Outport
  wires:
  rd_addr/1 -> Simple Dual Port RAM/4(rd_addr)
  wr_en/1 -> Simple Dual Port RAM/3(wr_en)
  wr_addr/1 -> Simple Dual Port RAM/2(wr_addr)
  wr_data/1 -> Simple Dual Port RAM/1(wr_data)
  Simple Dual Port RAM/1(rd_data) -> rd_data/1

== system gm_parallel_lht/Parallel LHT/Parallel LHT Accumulator/Accumulator with Switches/Accumulator_instance82/Block RAM ==
  wr_data : Inport  OutDataTypeStr=fixdt(0, 10, 0)  PortDimensions=1  SampleTime=6.66666666666667e-09
  wr_addr : Inport  Port=2  OutDataTypeStr=fixdt(0, 10, 0)  PortDimensions=1  SampleTime=6.66666666666667e-09
  wr_en : Inport  Port=3  OutDataTypeStr=boolean  PortDimensions=1  SampleTime=6.66666666666667e-09
  rd_addr : Inport  Port=4  OutDataTypeStr=fixdt(0, 10, 0)  PortDimensions=1  SampleTime=6.66666666666667e-09
  Simple Dual Port RAM : Subsystem
  rd_data : Outport
  wires:
  rd_addr/1 -> Simple Dual Port RAM/4(rd_addr)
  wr_en/1 -> Simple Dual Port RAM/3(wr_en)
  wr_addr/1 -> Simple Dual Port RAM/2(wr_addr)
  wr_data/1 -> Simple Dual Port RAM/1(wr_data)
  Simple Dual Port RAM/1(rd_data) -> rd_data/1

== system gm_parallel_lht/Parallel LHT/Parallel LHT Accumulator/Accumulator with Switches/Accumulator_instance83/Block RAM ==
  wr_data : Inport  OutDataTypeStr=fixdt(0, 10, 0)  PortDimensions=1  SampleTime=6.66666666666667e-09
  wr_addr : Inport  Port=2  OutDataTypeStr=fixdt(0, 10, 0)  PortDimensions=1  SampleTime=6.66666666666667e-09
  wr_en : Inport  Port=3  OutDataTypeStr=boolean  PortDimensions=1  SampleTime=6.66666666666667e-09
  rd_addr : Inport  Port=4  OutDataTypeStr=fixdt(0, 10, 0)  PortDimensions=1  SampleTime=6.66666666666667e-09
  Simple Dual Port RAM : Subsystem
  rd_data : Outport
  wires:
  rd_addr/1 -> Simple Dual Port RAM/4(rd_addr)
  wr_en/1 -> Simple Dual Port RAM/3(wr_en)
  wr_addr/1 -> Simple Dual Port RAM/2(wr_addr)
  wr_data/1 -> Simple Dual Port RAM/1(wr_data)
  Simple Dual Port RAM/1(rd_data) -> rd_data/1

== system gm_parallel_lht/Parallel LHT/Parallel LHT Accumulator/Accumulator with Switches/Accumulator_instance84/Block RAM ==
  wr_data : Inport  OutDataTypeStr=fixdt(0, 10, 0)  PortDimensions=1  SampleTime=6.66666666666667e-09
  wr_addr : Inport  Port=2  OutDataTypeStr=fixdt(0, 10, 0)  PortDimensions=1  SampleTime=6.66666666666667e-09
  wr_en : Inport  Port=3  OutDataTypeStr=boolean  PortDimensions=1  SampleTime=6.66666666666667e-09
  rd_addr : Inport  Port=4  OutDataTypeStr=fixdt(0, 10, 0)  PortDimensions=1  SampleTime=6.66666666666667e-09
  Simple Dual Port RAM : Subsystem
  rd_data : Outport
  wires:
  rd_addr/1 -> Simple Dual Port RAM/4(rd_addr)
  wr_en/1 -> Simple Dual Port RAM/3(wr_en)
  wr_addr/1 -> Simple Dual Port RAM/2(wr_addr)
  wr_data/1 -> Simple Dual Port RAM/1(wr_data)
  Simple Dual Port RAM/1(rd_data) -> rd_data/1

== system gm_parallel_lht/Parallel LHT/Parallel LHT Accumulator/Accumulator with Switches/Accumulator_instance85/Block RAM ==
  wr_data : Inport  OutDataTypeStr=fixdt(0, 10, 0)  PortDimensions=1  SampleTime=6.66666666666667e-09
  wr_addr : Inport  Port=2  OutDataTypeStr=fixdt(0, 10, 0)  PortDimensions=1  SampleTime=6.66666666666667e-09
  wr_en : Inport  Port=3  OutDataTypeStr=boolean  PortDimensions=1  SampleTime=6.66666666666667e-09
  rd_addr : Inport  Port=4  OutDataTypeStr=fixdt(0, 10, 0)  PortDimensions=1  SampleTime=6.66666666666667e-09
  Simple Dual Port RAM : Subsystem
  rd_data : Outport
  wires:
  rd_addr/1 -> Simple Dual Port RAM/4(rd_addr)
  wr_en/1 -> Simple Dual Port RAM/3(wr_en)
  wr_addr/1 -> Simple Dual Port RAM/2(wr_addr)
  wr_data/1 -> Simple Dual Port RAM/1(wr_data)
  Simple Dual Port RAM/1(rd_data) -> rd_data/1

== system gm_parallel_lht/Parallel LHT/Parallel LHT Accumulator/Accumulator with Switches/Accumulator_instance86/Block RAM ==
  wr_data : Inport  OutDataTypeStr=fixdt(0, 10, 0)  PortDimensions=1  SampleTime=6.66666666666667e-09
  wr_addr : Inport  Port=2  OutDataTypeStr=fixdt(0, 10, 0)  PortDimensions=1  SampleTime=6.66666666666667e-09
  wr_en : Inport  Port=3  OutDataTypeStr=boolean  PortDimensions=1  SampleTime=6.66666666666667e-09
  rd_addr : Inport  Port=4  OutDataTypeStr=fixdt(0, 10, 0)  PortDimensions=1  SampleTime=6.66666666666667e-09
  Simple Dual Port RAM : Subsystem
  rd_data : Outport
  wires:
  rd_addr/1 -> Simple Dual Port RAM/4(rd_addr)
  wr_en/1 -> Simple Dual Port RAM/3(wr_en)
  wr_addr/1 -> Simple Dual Port RAM/2(wr_addr)
  wr_data/1 -> Simple Dual Port RAM/1(wr_data)
  Simple Dual Port RAM/1(rd_data) -> rd_data/1

== system gm_parallel_lht/Parallel LHT/Parallel LHT Accumulator/Accumulator with Switches/Accumulator_instance87/Block RAM ==
  wr_data : Inport  OutDataTypeStr=fixdt(0, 10, 0)  PortDimensions=1  SampleTime=6.66666666666667e-09
  wr_addr : Inport  Port=2  OutDataTypeStr=fixdt(0, 10, 0)  PortDimensions=1  SampleTime=6.66666666666667e-09
  wr_en : Inport  Port=3  OutDataTypeStr=boolean  PortDimensions=1  SampleTime=6.66666666666667e-09
  rd_addr : Inport  Port=4  OutDataTypeStr=fixdt(0, 10, 0)  PortDimensions=1  SampleTime=6.66666666666667e-09
  Simple Dual Port RAM : Subsystem
  rd_data : Outport
  wires:
  rd_addr/1 -> Simple Dual Port RAM/4(rd_addr)
  wr_en/1 -> Simple Dual Port RAM/3(wr_en)
  wr_addr/1 -> Simple Dual Port RAM/2(wr_addr)
  wr_data/1 -> Simple Dual Port RAM/1(wr_data)
  Simple Dual Port RAM/1(rd_data) -> rd_data/1

== system gm_parallel_lht/Parallel LHT/Parallel LHT Accumulator/Accumulator with Switches/Accumulator_instance88/Block RAM ==
  wr_data : Inport  OutDataTypeStr=fixdt(0, 10, 0)  PortDimensions=1  SampleTime=6.66666666666667e-09
  wr_addr : Inport  Port=2  OutDataTypeStr=fixdt(0, 10, 0)  PortDimensions=1  SampleTime=6.66666666666667e-09
  wr_en : Inport  Port=3  OutDataTypeStr=boolean  PortDimensions=1  SampleTime=6.66666666666667e-09
  rd_addr : Inport  Port=4  OutDataTypeStr=fixdt(0, 10, 0)  PortDimensions=1  SampleTime=6.66666666666667e-09
  Simple Dual Port RAM : Subsystem
  rd_data : Outport
  wires:
  rd_addr/1 -> Simple Dual Port RAM/4(rd_addr)
  wr_en/1 -> Simple Dual Port RAM/3(wr_en)
  wr_addr/1 -> Simple Dual Port RAM/2(wr_addr)
  wr_data/1 -> Simple Dual Port RAM/1(wr_data)
  Simple Dual Port RAM/1(rd_data) -> rd_data/1

== system gm_parallel_lht/Parallel LHT/Parallel LHT Accumulator/Accumulator with Switches/Accumulator_instance89/Block RAM ==
  wr_data : Inport  OutDataTypeStr=fixdt(0, 10, 0)  PortDimensions=1  SampleTime=6.66666666666667e-09
  wr_addr : Inport  Port=2  OutDataTypeStr=fixdt(0, 10, 0)  PortDimensions=1  SampleTime=6.66666666666667e-09
  wr_en : Inport  Port=3  OutDataTypeStr=boolean  PortDimensions=1  SampleTime=6.66666666666667e-09
  rd_addr : Inport  Port=4  OutDataTypeStr=fixdt(0, 10, 0)  PortDimensions=1  SampleTime=6.66666666666667e-09
  Simple Dual Port RAM : Subsystem
  rd_data : Outport
  wires:
  rd_addr/1 -> Simple Dual Port RAM/4(rd_addr)
  wr_en/1 -> Simple Dual Port RAM/3(wr_en)
  wr_addr/1 -> Simple Dual Port RAM/2(wr_addr)
  wr_data/1 -> Simple Dual Port RAM/1(wr_data)
  Simple Dual Port RAM/1(rd_data) -> rd_data/1

== system gm_parallel_lht/Parallel LHT/Parallel LHT Accumulator/Accumulator with Switches/Accumulator_instance9/Block RAM ==
  wr_data : Inport  OutDataTypeStr=fixdt(0, 10, 0)  PortDimensions=1  SampleTime=6.66666666666667e-09
  wr_addr : Inport  Port=2  OutDataTypeStr=fixdt(0, 10, 0)  PortDimensions=1  SampleTime=6.66666666666667e-09
  wr_en : Inport  Port=3  OutDataTypeStr=boolean  PortDimensions=1  SampleTime=6.66666666666667e-09
  rd_addr : Inport  Port=4  OutDataTypeStr=fixdt(0, 10, 0)  PortDimensions=1  SampleTime=6.66666666666667e-09
  Simple Dual Port RAM : Subsystem
  rd_data : Outport
  wires:
  rd_addr/1 -> Simple Dual Port RAM/4(rd_addr)
  wr_en/1 -> Simple Dual Port RAM/3(wr_en)
  wr_addr/1 -> Simple Dual Port RAM/2(wr_addr)
  wr_data/1 -> Simple Dual Port RAM/1(wr_data)
  Simple Dual Port RAM/1(rd_data) -> rd_data/1

== system gm_parallel_lht/Parallel LHT/Parallel LHT Accumulator/Accumulator with Switches/Accumulator_instance90/Block RAM ==
  wr_data : Inport  OutDataTypeStr=fixdt(0, 10, 0)  PortDimensions=1  SampleTime=6.66666666666667e-09
  wr_addr : Inport  Port=2  OutDataTypeStr=fixdt(0, 10, 0)  PortDimensions=1  SampleTime=6.66666666666667e-09
  wr_en : Inport  Port=3  OutDataTypeStr=boolean  PortDimensions=1  SampleTime=6.66666666666667e-09
  rd_addr : Inport  Port=4  OutDataTypeStr=fixdt(0, 10, 0)  PortDimensions=1  SampleTime=6.66666666666667e-09
  Simple Dual Port RAM : Subsystem
  rd_data : Outport
  wires:
  rd_addr/1 -> Simple Dual Port RAM/4(rd_addr)
  wr_en/1 -> Simple Dual Port RAM/3(wr_en)
  wr_addr/1 -> Simple Dual Port RAM/2(wr_addr)
  wr_data/1 -> Simple Dual Port RAM/1(wr_data)
  Simple Dual Port RAM/1(rd_data) -> rd_data/1

== system gm_parallel_lht/Parallel LHT/Parallel LHT Accumulator/Accumulator with Switches/Accumulator_instance91/Block RAM ==
  wr_data : Inport  OutDataTypeStr=fixdt(0, 10, 0)  PortDimensions=1  SampleTime=6.66666666666667e-09
  wr_addr : Inport  Port=2  OutDataTypeStr=fixdt(0, 10, 0)  PortDimensions=1  SampleTime=6.66666666666667e-09
  wr_en : Inport  Port=3  OutDataTypeStr=boolean  PortDimensions=1  SampleTime=6.66666666666667e-09
  rd_addr : Inport  Port=4  OutDataTypeStr=fixdt(0, 10, 0)  PortDimensions=1  SampleTime=6.66666666666667e-09
  Simple Dual Port RAM : Subsystem
  rd_data : Outport
  wires:
  rd_addr/1 -> Simple Dual Port RAM/4(rd_addr)
  wr_en/1 -> Simple Dual Port RAM/3(wr_en)
  wr_addr/1 -> Simple Dual Port RAM/2(wr_addr)
  wr_data/1 -> Simple Dual Port RAM/1(wr_data)
  Simple Dual Port RAM/1(rd_data) -> rd_data/1

== system gm_parallel_lht/Parallel LHT/Parallel LHT Accumulator/Accumulator with Switches/Accumulator_instance92/Block RAM ==
  wr_data : Inport  OutDataTypeStr=fixdt(0, 10, 0)  PortDimensions=1  SampleTime=6.66666666666667e-09
  wr_addr : Inport  Port=2  OutDataTypeStr=fixdt(0, 10, 0)  PortDimensions=1  SampleTime=6.66666666666667e-09
  wr_en : Inport  Port=3  OutDataTypeStr=boolean  PortDimensions=1  SampleTime=6.66666666666667e-09
  rd_addr : Inport  Port=4  OutDataTypeStr=fixdt(0, 10, 0)  PortDimensions=1  SampleTime=6.66666666666667e-09
  Simple Dual Port RAM : Subsystem
  rd_data : Outport
  wires:
  rd_addr/1 -> Simple Dual Port RAM/4(rd_addr)
  wr_en/1 -> Simple Dual Port RAM/3(wr_en)
  wr_addr/1 -> Simple Dual Port RAM/2(wr_addr)
  wr_data/1 -> Simple Dual Port RAM/1(wr_data)
  Simple Dual Port RAM/1(rd_data) -> rd_data/1

== system gm_parallel_lht/Parallel LHT/Parallel LHT Accumulator/Accumulator with Switches/Accumulator_instance93/Block RAM ==
  wr_data : Inport  OutDataTypeStr=fixdt(0, 10, 0)  PortDimensions=1  SampleTime=6.66666666666667e-09
  wr_addr : Inport  Port=2  OutDataTypeStr=fixdt(0, 10, 0)  PortDimensions=1  SampleTime=6.66666666666667e-09
  wr_en : Inport  Port=3  OutDataTypeStr=boolean  PortDimensions=1  SampleTime=6.66666666666667e-09
  rd_addr : Inport  Port=4  OutDataTypeStr=fixdt(0, 10, 0)  PortDimensions=1  SampleTime=6.66666666666667e-09
  Simple Dual Port RAM : Subsystem
  rd_data : Outport
  wires:
  rd_addr/1 -> Simple Dual Port RAM/4(rd_addr)
  wr_en/1 -> Simple Dual Port RAM/3(wr_en)
  wr_addr/1 -> Simple Dual Port RAM/2(wr_addr)
  wr_data/1 -> Simple Dual Port RAM/1(wr_data)
  Simple Dual Port RAM/1(rd_data) -> rd_data/1
